simulink model "simu_sat"  (R2018b)
settings: Solver=FixedStepAuto  StartTime=0.0  StopTime=0.2  FixedStep=0.0001  RelTol=1e-3
settings Model: Creator=lubuntu  LastModifiedBy=lubuntu

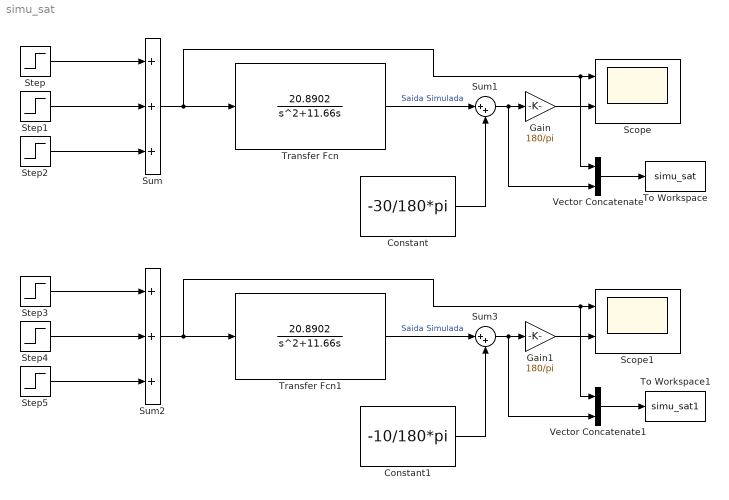
== system simu_sat ==
  Constant : Constant  Value=-30/180*pi
  Constant1 : Constant  Value=-10/180*pi
  Gain : Gain  Gain=180/pi
  Gain1 : Gain  Gain=180/pi
  Scope : Scope  NumInputPorts=2
  Scope1 : Scope  NumInputPorts=2
  Step : Step  Time=0.1  After=7  SampleTime=0
  Step1 : Step  Time=0.233  After=-14  SampleTime=0
  Step2 : Step  Time=0.283  After=7  SampleTime=0
  Step3 : Step  Time=0.05  After=7  SampleTime=0
  Step4 : Step  Time=0.114  After=-14  SampleTime=0
  Step5 : Step  Time=0.150  After=7  SampleTime=0
  Sum : Sum  Inputs=+++
  Sum1 : Sum  Inputs=|++
  Sum2 : Sum  Inputs=+++
  Sum3 : Sum  Inputs=|++
  To Workspace : ToWorkspace  VariableName=simu_sat  SaveFormat=Timeseries  SampleTime=-1
  To Workspace1 : ToWorkspace  VariableName=simu_sat1  SaveFormat=Timeseries  SampleTime=-1
  Transfer Fcn : TransferFcn  Numerator=[ 20.8902 ]  Denominator=[1 11.66 0]
  Transfer Fcn1 : TransferFcn  Numerator=[ 20.8902 ]  Denominator=[1 11.66 0]
  Vector Concatenate : Concatenate
  Vector Concatenate1 : Concatenate
  wires:
  Sum/1 -> Vector Concatenate/1, Scope/1, Transfer Fcn/1
  Step/1 -> Sum/1
  Step1/1 -> Sum/2
  Transfer Fcn/1 -> Sum1/1  "Saida Simulada"
  Sum1/1 -> Vector Concatenate/2, Gain/1
  Constant/1 -> Sum1/2
  Gain/1 -> Scope/2
  Step2/1 -> Sum/3
  Vector Concatenate/1 -> To Workspace/1
  Vector Concatenate1/1 -> To Workspace1/1
  Constant1/1 -> Sum3/2
  Transfer Fcn1/1 -> Sum3/1  "Saida Simulada"
  Sum3/1 -> Vector Concatenate1/2, Gain1/1
  Gain1/1 -> Scope1/2
  Step5/1 -> Sum2/3
  Step4/1 -> Sum2/2
  Sum2/1 -> Vector Concatenate1/1, Scope1/1, Transfer Fcn1/1
  Step3/1 -> Sum2/1
